simulink model "LongDendriteCells2"  (Simulink 10.2)
settings: Solver=ode45  StartTime=0.0  StopTime=1.5  RelTol=1e-3  EnableMultiTasking=on
libraries: NeuroModelerLibrary x10
settings Model: Creator=Bakhshiev  LastModifiedBy=Bakhshiev
settings SolverCC: ZeroCrossAlgorithm=Non-adaptive
settings DataIOCC: LimitDataPoints=on
settings OptimizationCC: ExpressionDepthLimit=2147483647  InitFltsAndDblsToZero=on
settings DebuggingCC: SolverPrmCheckMsg=warning  StateNameClashWarn=warning
settings SFSimCC: SimUseLocalCustomCode=on  CustomCodeUndefinedFunction=FilterOut
settings RTWCC: RTWUseLocalCustomCode=on
settings ConfigComp: CovExternalEMLEnable=on

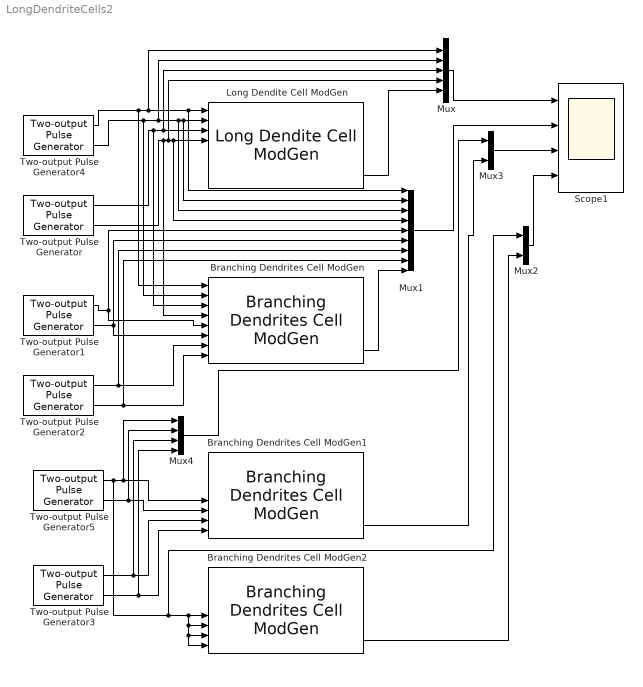
== system LongDendriteCells2 ==
  Branching Dendrites Cell ModGen : NeuroModelerLibrary/Dendrites Cells/Branching Dendrites Cell ModGen  SystemSampleTime=-1  VariantActivationTime=update diagram  Latency=0  AutoFrameSizeCalculation=off
  Branching Dendrites Cell ModGen1 : NeuroModelerLibrary/Dendrites Cells/Branching Dendrites Cell ModGen  SystemSampleTime=-1  VariantActivationTime=update diagram  Latency=0  AutoFrameSizeCalculation=off
  Branching Dendrites Cell ModGen2 : NeuroModelerLibrary/Dendrites Cells/Branching Dendrites Cell ModGen  SystemSampleTime=-1  VariantActivationTime=update diagram  Latency=0  AutoFrameSizeCalculation=off
  Long Dendite Cell ModGen : NeuroModelerLibrary/Dendrites Cells/Long Dendite Cell ModGen  SystemSampleTime=-1  VariantActivationTime=update diagram  Latency=0  AutoFrameSizeCalculation=off
  Mux : Mux  Inputs=5
  Mux1 : Mux  Inputs=9
  Mux2 : Mux  Inputs=2
  Mux3 : Mux  Inputs=2
  Mux4 : Mux
  Scope1 : Scope  NumInputPorts=4
  Two-output Pulse Generator : NeuroModelerLibrary/Support/Two-output Pulse Generator  A=1  P1=200  P2=200  PW=1  ST=0.001  OOn1=0.9  OOff1=1.0  OOn2=1.1  OOff2=1.2
  Two-output Pulse Generator1 : NeuroModelerLibrary/Support/Two-output Pulse Generator  A=1  P1=200  P2=200  PW=1  ST=0.001  OOn1=0.55  OOff1=0.6  OOn2=0.72  OOff2=0.8
  Two-output Pulse Generator2 : NeuroModelerLibrary/Support/Two-output Pulse Generator  A=1  P1=200  P2=200  PW=1  ST=0.001  OOn1=0.95  OOff1=1.1  OOn2=1.12  OOff2=1.2
  Two-output Pulse Generator3 : NeuroModelerLibrary/Support/Two-output Pulse Generator  A=1  P1=200  P2=200  PW=1  ST=0.001  OOn1=0.6  OOff1=0.7  OOn2=0.65  OOff2=0.7
  Two-output Pulse Generator4 : NeuroModelerLibrary/Support/Two-output Pulse Generator  A=1  P1=200  P2=200  PW=1  ST=0.001  OOn1=0.5  OOff1=0.6  OOn2=0.7  OOff2=0.8
  Two-output Pulse Generator5 : NeuroModelerLibrary/Support/Two-output Pulse Generator  A=1  P1=200  P2=200  PW=1  ST=0.001  OOn1=0.5  OOff1=0.6  OOn2=0.55  OOff2=0.6
  wires:
  Two-output Pulse Generator4/1 -> Branching Dendrites Cell ModGen/1, Mux/1, Long Dendite Cell ModGen/1, Mux1/1
  Two-output Pulse Generator4/2 -> Branching Dendrites Cell ModGen/2, Mux/2, Long Dendite Cell ModGen/2, Mux1/2, Mux1/3
  Mux/1 -> Scope1/1
  Two-output Pulse Generator/2 -> Branching Dendrites Cell ModGen/4, Mux/4, Long Dendite Cell ModGen/4, Mux1/4
  Two-output Pulse Generator/1 -> Branching Dendrites Cell ModGen/3, Long Dendite Cell ModGen/3, Mux/3
  Long Dendite Cell ModGen/3 -> Mux/5
  Two-output Pulse Generator1/1 -> Branching Dendrites Cell ModGen/5, Mux1/5
  Two-output Pulse Generator1/2 -> Branching Dendrites Cell ModGen/6, Mux1/6
  Two-output Pulse Generator2/1 -> Branching Dendrites Cell ModGen/7, Mux1/7
  Two-output Pulse Generator2/2 -> Branching Dendrites Cell ModGen/8, Mux1/8
  Two-output Pulse Generator5/1 -> Branching Dendrites Cell ModGen1/5, Mux4/1, Branching Dendrites Cell ModGen2/5, Branching Dendrites Cell ModGen2/6, Branching Dendrites Cell ModGen2/8, Branching Dendrites Cell ModGen2/7, Mux2/1
  Two-output Pulse Generator5/2 -> Branching Dendrites Cell ModGen1/6, Mux4/2
  Two-output Pulse Generator3/1 -> Branching Dendrites Cell ModGen1/7, Mux4/3
  Two-output Pulse Generator3/2 -> Branching Dendrites Cell ModGen1/8, Mux4/4
  Mux2/1 -> Scope1/4
  Branching Dendrites Cell ModGen2/3 -> Mux2/2
  Branching Dendrites Cell ModGen1/3 -> Mux3/2
  Branching Dendrites Cell ModGen/3 -> Mux1/9
  Mux1/1 -> Scope1/2
  Mux3/1 -> Scope1/3
  Mux4/1 -> Mux3/1
